simulink model "part3sim"  (R2025a)
settings: Solver=VariableStepAuto  StartTime=0.0  StopTime=5  RelTol=1e-3
values from neighbouring files (symbols this model uses):
  A = [ 0,       -1/L; 1/C,  -1/(R*C) ]    [PEproj3.m]
  B = [ uin/L; 0]    [PEproj3.m]
  C_mat = [0, 1]    [PEproj3.m]
  D = 0    [PEproj3.m]
undefined symbols (not defined in the file or in its folder): Ac, Bc, Cc, Dc
settings Model: Creator=Hp  LastModifiedBy=Hp

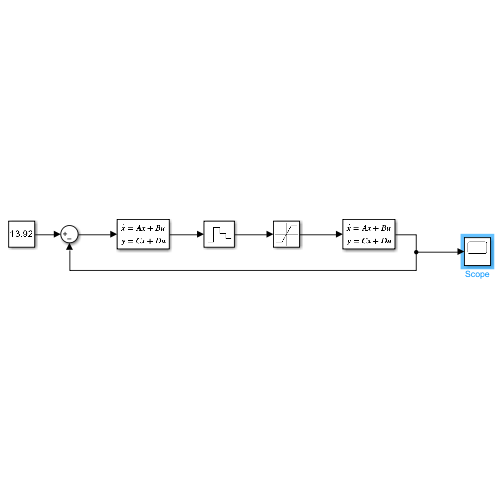
[thumbnail: Simulink's stored preview of the top-level diagram]
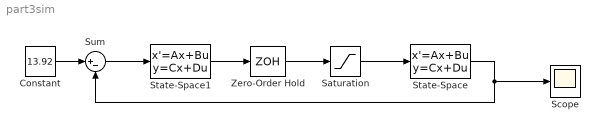
== system part3sim ==
  Constant : Constant  Value=13.92
  Saturation : Saturate  UpperLimit=1  LowerLimit=0
  Scope : Scope
      settings: ActiveDisplayYMinimum=13.919999295067202  ActiveDisplayYMaximum=13.920000643931049
  State-Space : StateSpace  A=A  B=B  C=C_mat  D=D  InitialCondition=0
  State-Space1 : StateSpace  A=Ac  B=Bc  C=Cc  D=Dc  InitialCondition=0
  Sum : Sum  Inputs=|+-
  Zero-Order Hold : ZeroOrderHold  SampleTime=1/(1500)
  wires:
  State-Space1/1 -> Zero-Order Hold/1
  Zero-Order Hold/1 -> Saturation/1
  Constant/1 -> Sum/1
  Saturation/1 -> State-Space/1
  State-Space/1 -> Sum/2, Scope/1
  Sum/1 -> State-Space1/1
